simulink model "math_model"  (R2020b)
settings: Solver=VariableStepAuto  StartTime=0.0  StopTime=10.0  RelTol=1e-3
settings Model: Creator=petir  LastModifiedBy=petir

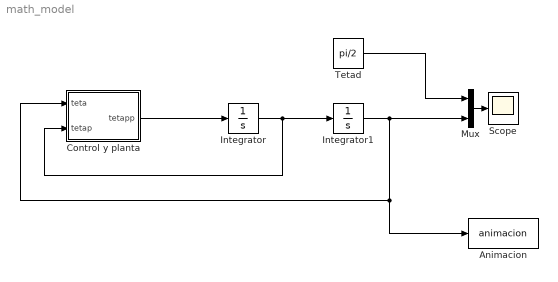
== system math_model ==
  Animacion : MATLABFcn  MATLABFcn=animacion  OutputDimensions=0
  Control y planta : MATLAB Function  TreatAsAtomicUnit=on
  Integrator : Integrator
  Integrator1 : Integrator
  Mux : Mux  Inputs=2
  Scope : Scope
  Tetad : Constant  Value=pi/2
  wires:
  Integrator/1 -> Control y planta/2(tetap), Integrator1/1
  Control y planta/1(tetapp) -> Integrator/1
  Integrator1/1 -> Animacion/1, Control y planta/1(teta), Mux/2
  Tetad/1 -> Mux/1
  Mux/1 -> Scope/1

== matlab function math_model/Control y planta ==
  data: teta input; tetapp output; tetap input
function tetapp = fcn(teta, tetap)
% Parametros
m = 1;
lc = 0.5;
I = 1;
g = 9.81;
B = 0.003;
kp = 450;
kd = 50;
tetad = pi / 2;

% Control
e =  tetad - teta;
tau  = kp * e - kd * tetap;

% Planta
tetapp = 1 / (m *lc^2 + I) * (tau - m*g*lc*sin(teta) - B*tetap);
